simulink model "dc_motor"  (Simulink 8.3)
settings: Solver=ode23tb  StartTime=0.0  StopTime=3.0  RelTol=1e-4
libraries: powerlib x11, powerlib_meascontrol x1
settings Model: Creator=zpwl83  LastModifiedBy=zpwl83
settings SolverCC: ZeroCrossAlgorithm=Adaptive
settings DataIOCC: SignalLoggingSaveFormat=Dataset
settings DebuggingCC: UnderspecifiedInitializationDetection=Simplified  StateNameClashWarn=none
settings GRTTargetCC: CombineOutputUpdateFcns=on  GRTInterface=off

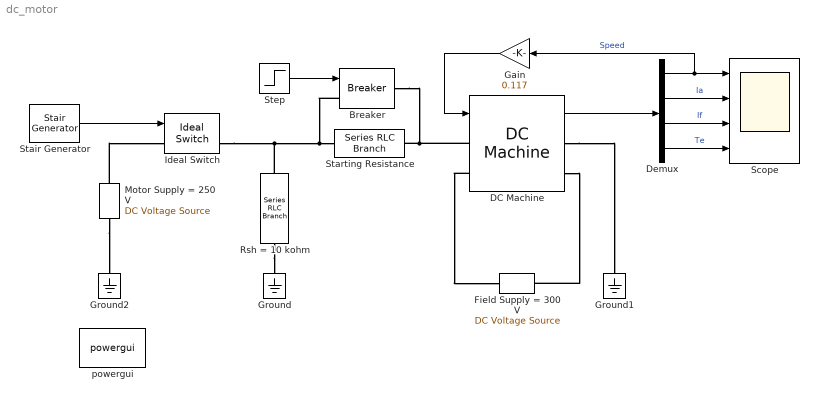
== system dc_motor ==
  Breaker : powerlib/Elements/Breaker  InitialState=0  SwitchingTimes="[1/60  5/60]"  External=on  BreakerResistance=0.01  SnubberResistance=1e6  SnubberCapacitance=inf  Measurements=None  MoreParameters=on  NoBreakLoop=off
  DC Machine : powerlib/Machines/DC Machine  PresetModel=01: 5HP 240V 1750RPM Field:300V  MechanicalLoad=Torque TL  FieldType=Wound  ShowDetailedParameters=on  MeasurementBus=off  RLa=[2.581 0.028]  RLf=[281.2 156]  Laf=0.9483  MachineConstant=Torque constant (N.m/A)  Ke=1.8  Kt=1.8  J=0.02215  Bm=0.002953  Tf=0.5161  w0=1  Ifinit=1  TsPowergui=0  TsBlock=-1
  Demux : Demux
  Field Supply = 300 V : powerlib/Electrical Sources/DC Voltage Source  Amplitude=300  Measurements=None
  Gain : Gain  Gain=0.117
  Ground : powerlib/Elements/Ground  LConnTagsString=a
  Ground1 : powerlib/Elements/Ground  LConnTagsString=a
  Ground2 : powerlib/Elements/Ground  LConnTagsString=a
  Ideal Switch : powerlib/Power Electronics/Ideal Switch  Ron=0.001  Lon=0  IC=0  Rs=1e5  Cs=inf  Measurements=on
  Motor Supply = 250 V : powerlib/Electrical Sources/DC Voltage Source  Amplitude=250  Measurements=None
  Rsh = 10 kohm : powerlib/Elements/Series RLC Branch  LConnTagsString=__new0  RConnTagsString=__new0  BranchType=R  Resistance=10000  Inductance=1e-3  SetiL0=off  InitialCurrent=0  Capacitance=1e-6  Setx0=off  InitialVoltage=0  Measurements=None
  Scope : Scope  NumInputPorts=4
      settings: YMin=-5~-5~-5~-5  YMax=5~5~5~5
  Stair Generator : powerlib_meascontrol/Pulse & Signal Generators/Stair Generator  t=[0, 0.5]  e=[0, 1]  Ts=0
  Starting Resistance : powerlib/Elements/Series RLC Branch  LConnTagsString=__new0  RConnTagsString=__new0  BranchType=R  Resistance=5.476  Inductance=1e-3  SetiL0=off  InitialCurrent=0  Capacitance=1e-6  Setx0=off  InitialVoltage=0  Measurements=None
  Step : Step  Time=2  SampleTime=0
  powergui : powerlib/powergui  Priority=1  SimulationMode=Continuous  SolverType=Tustin  SampleTime=50e-6  frequency=60  SPID=off  DisableSnubberDevices=off  DisableRonSwitches=off  DisableVfSwitches=off  SwTol=0  Interpol=off  DisplayEquations=off  Ts=0  methode=off  frequencyindice=0  Pbase=100e6  ErrMax=1e-4  Iterations=50  UnitsV=kV  UnitsW=MW  FunctionMessages=off  echomessages=off  HookPort=off  EnableUseOfTLC=off  x0status=blocks  RestoreLinks=warning  ResistiveCurrentMeasurement=off  Frange=[0:2:500]  Ylog=off  Xlog=on  ShowGrid=off  save=off  variable=ZData  structure=0  ZoomFFT=off  StartTime=0.0  cycles=1  DisplayStyle=1  fundamental=60  FreqAxis=off  MaxFrequency=1000  frequencyindicesteady=1  RmsSteady=1  display=off
  wires:
  Demux/1 -> Gain/1, Scope/1  "Speed"
  Demux/2 -> Scope/2  "Ia"
  Demux/3 -> Scope/3  "If"
  Demux/4 -> Scope/4  "Te"
  DC Machine/1 -> Demux/1
  Gain/1 -> DC Machine/1
  Step/1 -> Breaker/1
  Stair Generator/1 -> Ideal Switch/1
  connections:
  Breaker/RConn1 -- DC Machine/LConn1 -- Starting Resistance/RConn1
  Ideal Switch/RConn1 -- Rsh = 10 kohm/RConn1 -- Breaker/LConn1 -- Starting Resistance/LConn1
  Rsh = 10 kohm/LConn1 -- Ground/LConn1
  DC Machine/RConn1 -- Ground1/LConn1
  Motor Supply = 250 V/RConn1 -- Ideal Switch/LConn1
  Motor Supply = 250 V/LConn1 -- Ground2/LConn1
  DC Machine/LConn2 -- Field Supply = 300 V/RConn1
  DC Machine/RConn2 -- Field Supply = 300 V/LConn1
